simulink model "Hover_Simulink"  (R2025a)
settings: Solver=VariableStepAuto  StartTime=0.0  StopTime=90  RelTol=1e-3
libraries: SignalEditorBlockLib x1
settings Model: Creator=asing  LastModifiedBy=asing

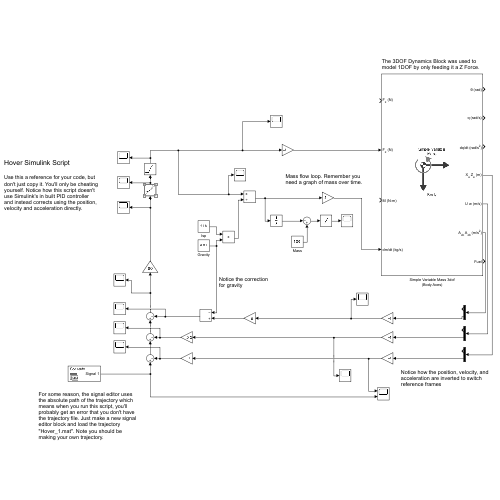
[thumbnail: Simulink's stored preview of the top-level diagram]
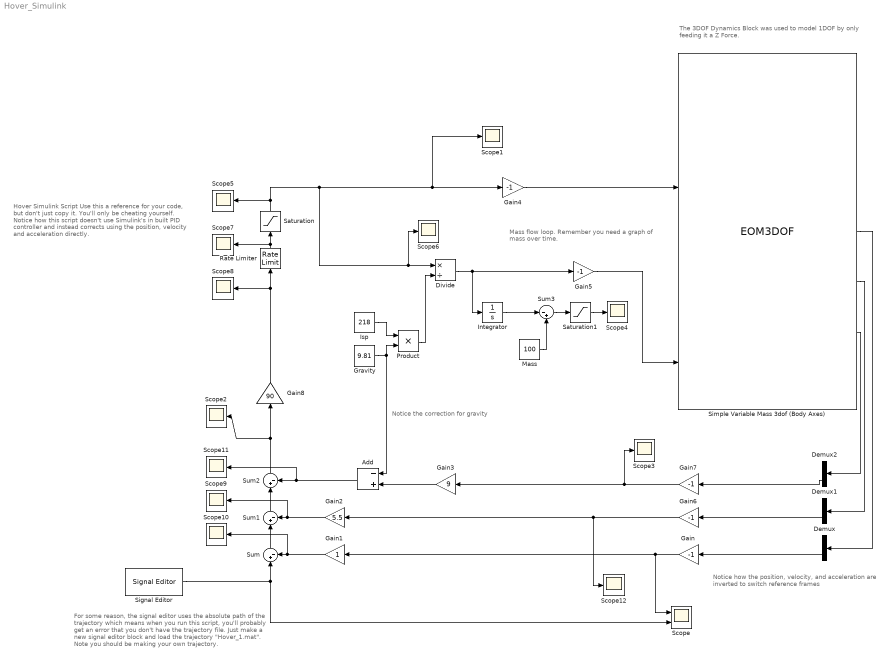
== system Hover_Simulink ==
  note: For some reason, the signal editor uses the absolute path of the trajectory which means when you run this script, you'll probably get an error that you don't have the trajectory file. Just make a new signal editor block and load the trajectory "Hover_1.mat". Note you should be making your own trajectory.
  note: Hover Simulink Script
      |
      | Use this a reference for your code, but don't just copy it. You'll only be cheating yourself. Notice how this script doesn't use Simulink's in built PID controller and instead corrects using the position, velocity and acceleration directly.
  note: The 3DOF Dynamics Block was used to model 1DOF by only feeding it a Z Force.
  note: Notice how the position, velocity, and acceleration are inverted to switch reference frames
  note: Notice the correction for gravity
  note: Mass flow loop. Remember you need a graph of mass over time.
  Add : Sum  Inputs=-+
  Demux : Demux  Outputs=2
  Demux1 : Demux  Outputs=2
  Demux2 : Demux  Outputs=2
  Divide : Product  Inputs=*/
  Gain{,4..7} (5 alike) : Gain  Gain=-1
  Gain1 : Gain
  Gain2 : Gain  Gain=5.5
  Gain3 : Gain  Gain=9
  Gain8 : Gain  Gain=90
  Gravity : Constant  Value=9.81
  Integrator : Integrator
  Isp : Constant  Value=218
  Mass : Constant  Value=100
  Product : Product
  Rate Limiter : RateLimiter  RisingSlewLimit=500  FallingSlewLimit=-500  SampleTimeMode=inherited
  Saturation : Saturate  UpperLimit=2400  LowerLimit=500  ZeroCross=off
  Saturation1 : Saturate  UpperLimit=100  LowerLimit=50
  Scope : Scope  NumInputPorts=2
      settings: ActiveDisplayYMinimum=18.89658413321229  ActiveDisplayYMaximum=40.821853322110471
  Scope{1..12} (12 alike) : Scope
      Scope1 settings: ActiveDisplayYMinimum=404.13461538461542  ActiveDisplayYMaximum=1362.7884615384614
      Scope10 settings: ActiveDisplayYMinimum=-1  ActiveDisplayYMaximum=1  DataLoggingVariableName=ScopeData10
      Scope11 settings: ActiveDisplayYMinimum=-47.394161296045475  ActiveDisplayYMaximum=38.633404117126219  DataLoggingVariableName=ScopeData11
      Scope12 settings: ActiveDisplayYMinimum=-17.386779443318023  ActiveDisplayYMaximum=14.310134554357177  DataLoggingVariableName=ScopeData12
      Scope2 settings: ActiveDisplayYMinimum=-58.600806341948541  ActiveDisplayYMaximum=88.817704094592486  DataLoggingVariableName=ScopeData2
      Scope3 settings: ActiveDisplayYMinimum=-53.073675047329495  ActiveDisplayYMaximum=78.859663187536924  DataLoggingVariableName=ScopeData3
      Scope4 settings: ActiveDisplayYMinimum=62.675720857132347  ActiveDisplayYMaximum=102.94357945039437  DataLoggingVariableName=ScopeData4
      Scope5 settings: ActiveDisplayYMinimum=262.50000000000006  ActiveDisplayYMaximum=2637.5  DataLoggingVariableName=ScopeData5
      Scope6 settings: ActiveDisplayYMinimum=-1  ActiveDisplayYMaximum=1  DataLoggingVariableName=ScopeData6
      Scope7 settings: ActiveDisplayYMinimum=-2229.2857142857156  ActiveDisplayYMaximum=3020.7142857142849  DataLoggingVariableName=ScopeData7
      Scope8 settings: ActiveDisplayYMinimum=-20583.369798983134  ActiveDisplayYMaximum=6330.7335301561079  DataLoggingVariableName=ScopeData8
      Scope9 settings: ActiveDisplayYMinimum=-95.627286938249114  ActiveDisplayYMaximum=78.705740048964458  DataLoggingVariableName=ScopeData9
  Signal Editor : SignalEditorBlockLib/Signal Editor  FileName=Hover_1.mat  ActiveScenario=Scenario  ActiveSignal=Signal 1  IsBus=off  OutputBusObjectStr=Bus: BusObject  SampleTime=0  ZeroCross=off  OutputAfterFinalValue=Setting to zero  Unit=inherit  PreserveSignalName=on  ApplySigPropsToAllScenarios=on  ApplySigPropsToAllSignals=off  SignalPropertySource=Dialog parameters
  Simple Variable Mass 3dof (Body Axes) : EOM3DOF  mtype=Simple Variable  v_ini=0  mass=100  mass_e=50  mass_f=100  Iyy_e=2500  Iyy_f=5000
  Sum : Sum  Inputs=|+-
  Sum1 : Sum  Inputs=|+-
  Sum2 : Sum  Inputs=|+-
  Sum3 : Sum  Inputs=|-+
  wires:
  Signal Editor/1 -> Scope/2, Sum/1
  Simple Variable Mass 3dof (Body Axes)/4 -> Demux/1
  Demux/2 -> Gain/1
  Gain/1 -> Scope/1, Gain1/1
  Sum/1 -> Sum1/1
  Sum1/1 -> Sum2/1
  Gain1/1 -> Scope10/1, Sum/2
  Simple Variable Mass 3dof (Body Axes)/5 -> Demux1/1
  Simple Variable Mass 3dof (Body Axes)/6 -> Demux2/1
  Demux1/2 -> Gain6/1
  Gain2/1 -> Scope9/1, Sum1/2
  Gain4/1 -> Simple Variable Mass 3dof (Body Axes)/2
  Rate Limiter/1 -> Saturation/1, Scope7/1
  Demux2/2 -> Gain7/1
  Isp/1 -> Product/1
  Gravity/1 -> Add/1, Product/2
  Product/1 -> Divide/2
  Gain5/1 -> Simple Variable Mass 3dof (Body Axes)/4
  Divide/1 -> Integrator/1, Gain5/1
  Integrator/1 -> Sum3/1
  Sum3/1 -> Saturation1/1
  Mass/1 -> Sum3/2
  Sum2/1 -> Gain8/1, Scope2/1
  Saturation/1 -> Scope5/1, Gain4/1, Scope1/1, Scope6/1, Divide/1
  Gain6/1 -> Scope12/1, Gain2/1
  Gain7/1 -> Scope3/1, Gain3/1
  Gain8/1 -> Scope8/1, Rate Limiter/1
  Gain3/1 -> Add/2
  Add/1 -> Scope11/1, Sum2/2
  Saturation1/1 -> Scope4/1
